simulink model "test_SYSTEME_ZIGBEE_2017"  (R2014b)
settings: Solver=ode45  SolverMode=SingleTasking  StartTime=0.0  StopTime=1E-3  RelTol=1e-3
libraries: dspsrcs4 x8, dsparch4 x7, simulink x3, dspstat3 x2, commsink2 x1, commrandsrc2 x1, commdigbbndcpm2 x1, simulink_extras x1, dspsigops x1
settings Model: DisableUpgradeWarningsForVersion=R2015a  CovSFcnEnable=on  Creator=Yannis  LastModifiedBy=xph2app003
settings OptimizationCC: BlockReduction=off  BooleanDataType=off
settings DebuggingCC: SaveWithParameterizedLinksMsg=none  UnderspecifiedInitializationDetection=Classic  MergeDetectMultiDrivingBlocksExec=none  SignalResolutionControl=TryResolveAllWithWarning  SolverPrmCheckMsg=none
settings HardwareCC: TargetBitPerLong=64  TargetBitPerPointer=64  TargetLongLongMode=on  TargetIntDivRoundTo=Zero  TargetEndianess=LittleEndian  TargetWordSize=64  TargetHWDeviceType=MATLAB Host  ProdEqTarget=off

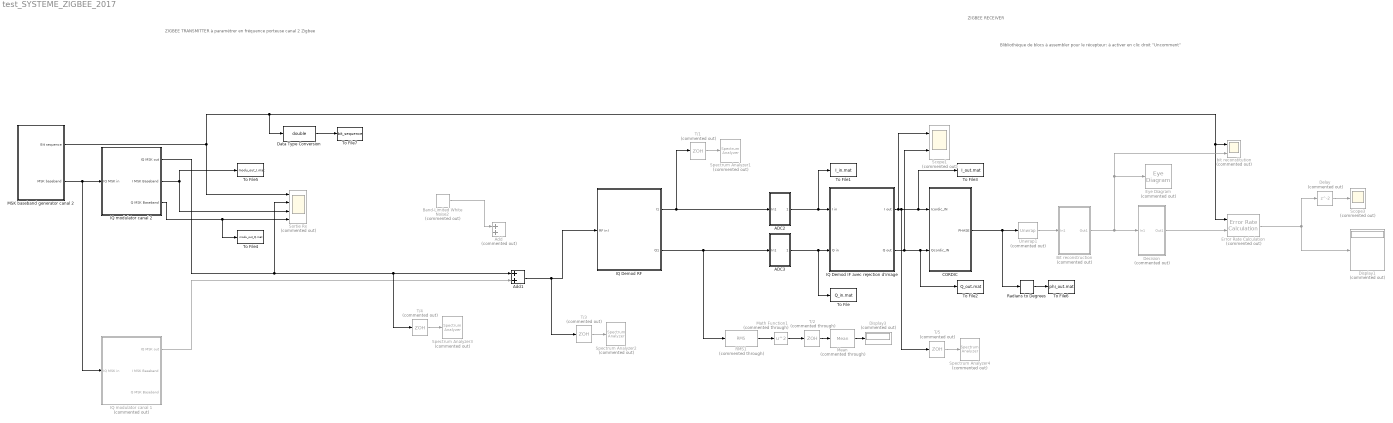
== system test_SYSTEME_ZIGBEE_2017 ==
  note: ZIGBEE RECEIVER
  note: ZIGBEE TRANSMITTER
      | à paramétrer en fréquence porteuse
      | canal 2  Zigbee
  note: Blibliothèque de blocs à assembler pour le récepteur: à activer en clic droit "Uncomment"
  ADC2 : Subsystem
  ADC3 : Subsystem
  Add : Sum  Commented=on
  Add1 : Sum
  Band-Limited White Noise2 : simulink/Sources/Band-Limited White Noise  Commented=on  Cov=[1e-9]  Ts=5e-10  seed=[23341]
  Bit reconstruction : Subsystem  Commented=on
  CORDIC : Subsystem
  Data Type Conversion : DataTypeConversion  OutDataTypeStr=double
  Decision : Subsystem  Commented=on
  Delay : Delay  Commented=on  InitialCondition=0
  Display1 : Display  Commented=on
  Display3 : Display  Commented=on
  Error Rate Calculation : commsink2/Error Rate Calculation  Commented=on  N=1  st_delay=1  cp_mode=Entire frame  subframe=[]  PMode=Port  WsName=ErrorVec  RsMode2=off  stop=off  numErr=100  maxBits=1e6
  Eye Diagram : EyeDiagram  Commented=on
  IQ Demod IF avec rejection d'image : Subsystem  TreatAsAtomicUnit=on
  IQ Demod RF : Subsystem  TreatAsAtomicUnit=on
  IQ modulator canal 1 : Subsystem  Commented=on
  IQ modulator canal 2 : Subsystem
  MSK baseband generator canal 2 : Subsystem
  Math Function1 : Math  Commented=through  Operator=square  SaturateOnIntegerOverflow=on
  Mean : dspstat3/Mean  Commented=through  run=on  reset_popup=None  InputProcessing=Columns as channels (frame based)  directionMode=Each column  dimension=1  treatSBRowAsCol=on  roiEnable=off  roiType=Rectangles  roiPortion=Entire ROI  roiOutput=Individual statistics for each ROI  roiFlag=off  outputDataTypeStr=Inherit: Same as accumulator  outputLastDataTypeStr=Inherit: Same as accumulator  outputMin=[]  outputMax=[]  roundingMode=Floor  overflowMode=off
  RMS1 : dspstat3/RMS  Commented=through  run=off  reset_popup=None  InputProcessing=Columns as channels (frame based)  directionMode=Entire input  dimension=1  treatSBRowAsCol=on
  Radians to Degrees : simulink_extras/Transformations/Radians to Degrees
  Scope1 : Scope  Commented=on  NumInputPorts=2
      settings: YMin=-1.5~-1.5  YMax=1.5~1.5  MaxDataPoints=20000
  Scope3 : Scope  Commented=on
      settings: TimeRange=9.999999999999999e-05  YMin=-1  YMax=1  SaveName=ScopeData2
  Sortie Rx : Scope  Commented=on  NumInputPorts=4
      settings: TimeRange=1e-05  YMin=-1~-1.5~-1~-1  YMax=2~1.5~1~1
  Spectrum Analyzer{1..4} (4 alike) : SpectrumAnalyzer  Commented=on
  T/{1,3..5} (4 alike) : ZeroOrderHold  Commented=on  SampleTime=1/(10e6)
  T/2 : ZeroOrderHold  Commented=through  SampleTime=1/(10e6)
  To File : ToFile  Filename=Q_in.mat
  To File1 : ToFile  Filename=I_in.mat
  To File2 : ToFile  Filename=Q_out.mat
  To File3 : ToFile  Filename=I_out.mat
  To File4 : ToFile  Filename=modu_out_Q.mat
  To File5 : ToFile  Filename=modu_out_I.mat
  To File6 : ToFile  Filename=phi_out.mat
  To File7 : ToFile  Filename=bit_sequence  MatrixName=bit
  Unwrap1 : dspsigops/Unwrap  Commented=on  tol=pi  InputProcessing=Columns as channels (frame based)  running=off
  bit reconstitution : Scope  Commented=on  NumInputPorts=2
      settings: TimeRange=1.049040685224839e-05  YMin=-0.2~-2  YMax=3~0.6  SaveName=ScopeData4
  wires:
  Delay/1 -> Scope3/1
  MSK baseband generator canal 2/1(Bit sequence) -> Data Type Conversion/1, Error Rate Calculation/1, bit reconstitution/1, Sortie Rx/1
  IQ modulator canal 2/3(Q MSK Baseband) -> To File4/1, Sortie Rx/4
  Error Rate Calculation/1 -> Display1/1, Delay/1
  ADC2/1(Out1) -> To File1/1, IQ Demod IF avec rejection d'image/1("I in ")
  ADC3/1(Out1) -> To File/1, IQ Demod IF avec rejection d'image/2("Q in ")
  IQ modulator canal 2/2(I MSK Baseband) -> Sortie Rx/3, To File5/1
  IQ Demod RF/1(I1) -> ADC2/1(In1), T/1/1
  IQ Demod RF/2("Q1 ") -> RMS1/1, ADC3/1(In1)
  IQ Demod IF avec rejection d'image/2(Q out) -> To File2/1, CORDIC/2(Qcordic_IN), Scope1/2
  CORDIC/1(PHASE) -> Radians to Degrees/1, Unwrap1/1
  Unwrap1/1 -> Bit reconstruction/1(In1)
  Bit reconstruction/1(Out1) -> Eye Diagram/1, bit reconstitution/2, Decision/1(In1)
  T/1/1 -> Spectrum Analyzer1/1
  Decision/1(Out1) -> Error Rate Calculation/2
  Band-Limited White Noise2/1 -> Add/1
  RMS1/1 -> Math Function1/1
  T/2/1 -> Mean/1
  Mean/1 -> Display3/1
  Math Function1/1 -> T/2/1
  MSK baseband generator canal 2/2(MSK baseband) -> IQ modulator canal 1/1(IQ MSK in), IQ modulator canal 2/1(IQ MSK in)
  IQ modulator canal 1/1("IQ MSK out ") -> Add1/2
  Add1/1 -> T/3/1, IQ Demod RF/1(RF in I)
  T/3/1 -> Spectrum Analyzer2/1
  IQ modulator canal 2/1("IQ MSK out ") -> Sortie Rx/2, T/4/1, Add1/1
  T/4/1 -> Spectrum Analyzer3/1
  IQ Demod IF avec rejection d'image/1(I out) -> To File3/1, CORDIC/1(Icordic_IN), T/5/1, Scope1/1
  T/5/1 -> Spectrum Analyzer4/1
  Data Type Conversion/1 -> To File7/1
  Radians to Degrees/1 -> To File6/1

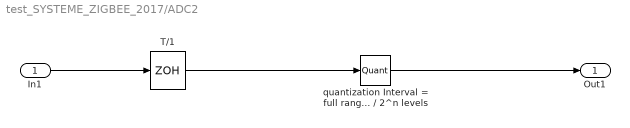
== system test_SYSTEME_ZIGBEE_2017/ADC2 ==
  In1 : Inport
  T/1 : ZeroOrderHold  SampleTime=1/(50e6)
  quantization Interval = full range (2Volts) / 2^n levels : Quantizer  QuantizationInterval=2/32  LinearizeAsGain=off  SampleTime=1/(50e6)
  Out1 : Outport
  wires:
  In1/1 -> T/1/1
  T/1/1 -> quantization Interval = full range (2Volts) / 2^n levels/1
  quantization Interval = full range (2Volts) / 2^n levels/1 -> Out1/1

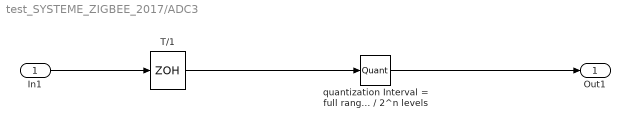
== system test_SYSTEME_ZIGBEE_2017/ADC3 ==
  In1 : Inport
  T/1 : ZeroOrderHold  SampleTime=1/(50e6)
  quantization Interval = full range (2Volts) / 2^n levels : Quantizer  QuantizationInterval=2/32  LinearizeAsGain=off  SampleTime=1/(50e6)
  Out1 : Outport
  wires:
  In1/1 -> T/1/1
  T/1/1 -> quantization Interval = full range (2Volts) / 2^n levels/1
  quantization Interval = full range (2Volts) / 2^n levels/1 -> Out1/1

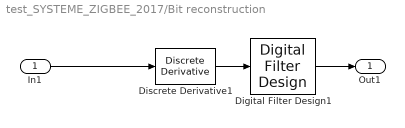
== system test_SYSTEME_ZIGBEE_2017/Bit reconstruction ==
  In1 : Inport
  Digital Filter Design1 : dsparch4/Digital Filter Design  mwdsp_browser_bugfix_var=off
  Discrete Derivative1 : simulink/Discrete/Discrete Derivative  gainval=1/(10e6)  ICPrevScaledInput=0.0  InputProcessing=Inherited  OutMin=[]  OutMax=[]  OutDataTypeStr=double  OutputDataTypeScalingMode=double  OutDataType=fixdt(1, 16)  OutScaling=2^-10  DoSatur=off
  Out1 : Outport
  wires:
  Discrete Derivative1/1 -> Digital Filter Design1/1
  Digital Filter Design1/1 -> Out1/1
  In1/1 -> Discrete Derivative1/1

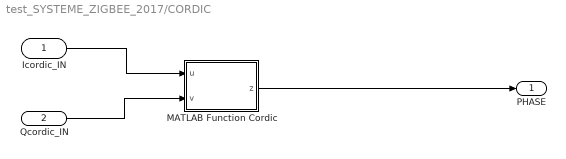
== system test_SYSTEME_ZIGBEE_2017/CORDIC ==
  Icordic_IN : Inport
  Qcordic_IN : Inport  Port=2
  MATLAB Function Cordic : MATLAB Function  TreatAsAtomicUnit=on
  PHASE : Outport
  wires:
  MATLAB Function Cordic/1(z) -> PHASE/1
  Icordic_IN/1 -> MATLAB Function Cordic/1(u)
  Qcordic_IN/1 -> MATLAB Function Cordic/2(v)

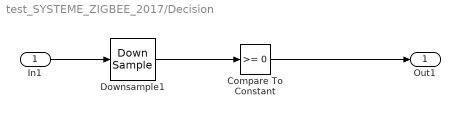
== system test_SYSTEME_ZIGBEE_2017/Decision ==
  In1 : Inport
  Compare To Constant : simulink/Logic and Bit Operations/Compare To Constant  relop=>=  const=0  OutDataTypeStr=boolean
  Downsample1 : DownSample  N=5  phase=2
  Out1 : Outport
  wires:
  Compare To Constant/1 -> Out1/1
  In1/1 -> Downsample1/1
  Downsample1/1 -> Compare To Constant/1

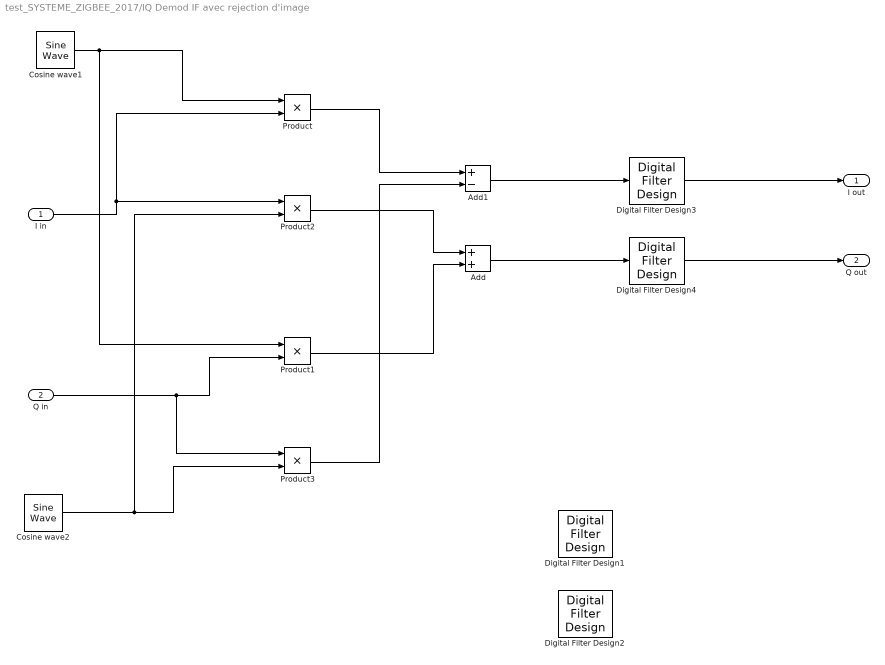
== system test_SYSTEME_ZIGBEE_2017/IQ Demod IF avec rejection d'image ==
  "I in " : Inport
  "Q in " : Inport  Port=2
  Add : Sum
  Add1 : Sum  Inputs=+-
  Cosine wave1 : dspsrcs4/Sine Wave  Amplitude=1  Frequency=2.5e6  Phase=pi/2  SampleMode=Discrete  OutComplex=Real  CompMethod=Trigonometric fcn  TableSize=Speed  SampleTime=1/(50e6)  SamplesPerFrame=1  ResetState=Restart at time zero  dataType=double  wordLen=16  udDataType=sfix(16)  fracBitsMode=Best precision  numFracBits=15  OutDataTypeStr=double  LastOutDataTypeStr=double
  Cosine wave2 : dspsrcs4/Sine Wave  Amplitude=1  Frequency=2.5e6  Phase=pi  SampleMode=Discrete  OutComplex=Real  CompMethod=Trigonometric fcn  TableSize=Speed  SampleTime=1/(50e6)  SamplesPerFrame=1  ResetState=Restart at time zero  dataType=double  wordLen=16  udDataType=sfix(16)  fracBitsMode=Best precision  numFracBits=15  OutDataTypeStr=double  LastOutDataTypeStr=double
  Digital Filter Design{1..4} (4 alike) : dsparch4/Digital Filter Design  mwdsp_browser_bugfix_var=off
  Product{,1..3} (4 alike) : Product
  I out : Outport
  Q out : Outport  Port=2
  wires:
  Cosine wave1/1 -> Product1/1, Product/1
  Cosine wave2/1 -> Product2/2, Product3/2
  "I in "/1 -> Product2/1, Product/2
  "Q in "/1 -> Product3/1, Product1/2
  Product/1 -> Add1/1
  Product3/1 -> Add1/2
  Product2/1 -> Add/1
  Product1/1 -> Add/2
  Add/1 -> Digital Filter Design4/1
  Digital Filter Design4/1 -> Q out/1
  Digital Filter Design3/1 -> I out/1
  Add1/1 -> Digital Filter Design3/1

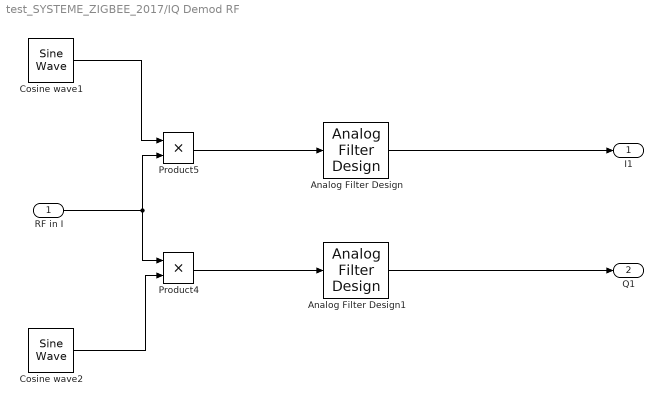
== system test_SYSTEME_ZIGBEE_2017/IQ Demod RF ==
  RF in I : Inport
  Analog Filter Design : dsparch4/Analog Filter Design  method=Butterworth  filttype=Lowpass  N=8  Wlo=31.4e6  Whi=80  Rp=2  Rs=40
  Analog Filter Design1 : dsparch4/Analog Filter Design  method=Butterworth  filttype=Lowpass  N=8  Wlo=31.4e6  Whi=80  Rp=2  Rs=40
  Cosine wave1 : dspsrcs4/Sine Wave  Amplitude=1  Frequency=2.4075e9  Phase=pi/2  SampleMode=Continuous  OutComplex=Real  CompMethod=Trigonometric fcn  TableSize=Speed  SampleTime=1/(10e6)  SamplesPerFrame=1  ResetState=Restart at time zero  dataType=double  wordLen=16  udDataType=sfix(16)  fracBitsMode=Best precision  numFracBits=15  OutDataTypeStr=double  LastOutDataTypeStr=double
  Cosine wave2 : dspsrcs4/Sine Wave  Amplitude=1  Frequency=2.4075e9  Phase=pi  SampleMode=Continuous  OutComplex=Real  CompMethod=Trigonometric fcn  TableSize=Speed  SampleTime=1/(10e6)  SamplesPerFrame=1  ResetState=Restart at time zero  dataType=double  wordLen=16  udDataType=sfix(16)  fracBitsMode=Best precision  numFracBits=15  OutDataTypeStr=double  LastOutDataTypeStr=double
  Product4 : Product  RndMeth=Zero
  Product5 : Product  RndMeth=Zero
  I1 : Outport
  "Q1 " : Outport  Port=2
  wires:
  RF in I/1 -> Product5/2, Product4/1
  Cosine wave2/1 -> Product4/2
  Cosine wave1/1 -> Product5/1
  Product5/1 -> Analog Filter Design/1
  Product4/1 -> Analog Filter Design1/1
  Analog Filter Design/1 -> I1/1
  Analog Filter Design1/1 -> "Q1 "/1

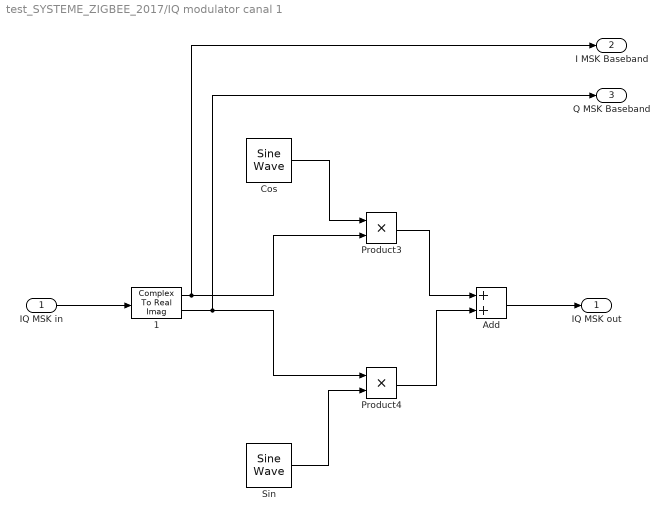
== system test_SYSTEME_ZIGBEE_2017/IQ modulator canal 1 ==
  IQ MSK in : Inport
  " 1" : ComplexToRealImag
  Add : Sum
  Cos : dspsrcs4/Sine Wave  Amplitude=1  Frequency=2.405e9  Phase=pi/2  SampleMode=Continuous  OutComplex=Real  CompMethod=Trigonometric fcn  TableSize=Speed  SampleTime=1/(8*2.4e9)  SamplesPerFrame=1  ResetState=Restart at time zero  dataType=double  wordLen=16  udDataType=sfix(16)  fracBitsMode=Best precision  numFracBits=15  OutDataTypeStr=double  LastOutDataTypeStr=double
  Product3 : Product  RndMeth=Zero
  Product4 : Product  RndMeth=Zero
  Sin : dspsrcs4/Sine Wave  Amplitude=1  Frequency=2.405E9  Phase=pi  SampleMode=Continuous  OutComplex=Real  CompMethod=Trigonometric fcn  TableSize=Speed  SampleTime=1/(4*2.4e9)  SamplesPerFrame=1  ResetState=Restart at time zero  dataType=double  wordLen=16  udDataType=sfix(16)  fracBitsMode=Best precision  numFracBits=15  OutDataTypeStr=double  LastOutDataTypeStr=double
  "IQ MSK out " : Outport
  I MSK Baseband : Outport  Port=2
  Q MSK Baseband : Outport  Port=3
  wires:
  Add/1 -> "IQ MSK out "/1
  Product4/1 -> Add/2
  " 1"/2 -> Product4/1, Q MSK Baseband/1
  " 1"/1 -> I MSK Baseband/1, Product3/2
  Sin/1 -> Product4/2
  Product3/1 -> Add/1
  Cos/1 -> Product3/1
  IQ MSK in/1 -> " 1"/1

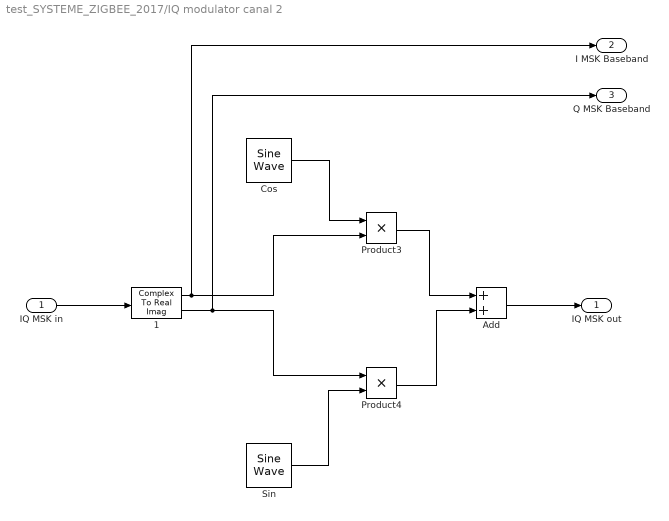
== system test_SYSTEME_ZIGBEE_2017/IQ modulator canal 2 ==
  IQ MSK in : Inport
  " 1" : ComplexToRealImag
  Add : Sum
  Cos : dspsrcs4/Sine Wave  Amplitude=1  Frequency=2.410e9  Phase=pi/2  SampleMode=Continuous  OutComplex=Real  CompMethod=Trigonometric fcn  TableSize=Speed  SampleTime=1/(8*2.4e9)  SamplesPerFrame=1  ResetState=Restart at time zero  dataType=double  wordLen=16  udDataType=sfix(16)  fracBitsMode=Best precision  numFracBits=15  OutDataTypeStr=double  LastOutDataTypeStr=double
  Product3 : Product  RndMeth=Zero
  Product4 : Product  RndMeth=Zero
  Sin : dspsrcs4/Sine Wave  Amplitude=1  Frequency=2.410E9  Phase=pi  SampleMode=Continuous  OutComplex=Real  CompMethod=Trigonometric fcn  TableSize=Speed  SampleTime=1/(4*2.4e9)  SamplesPerFrame=1  ResetState=Restart at time zero  dataType=double  wordLen=16  udDataType=sfix(16)  fracBitsMode=Best precision  numFracBits=15  OutDataTypeStr=double  LastOutDataTypeStr=double
  "IQ MSK out " : Outport
  I MSK Baseband : Outport  Port=2
  Q MSK Baseband : Outport  Port=3
  wires:
  Add/1 -> "IQ MSK out "/1
  Product4/1 -> Add/2
  " 1"/2 -> Product4/1, Q MSK Baseband/1
  " 1"/1 -> I MSK Baseband/1, Product3/2
  Sin/1 -> Product4/2
  Product3/1 -> Add/1
  Cos/1 -> Product3/1
  IQ MSK in/1 -> " 1"/1

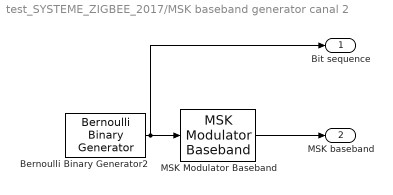
== system test_SYSTEME_ZIGBEE_2017/MSK baseband generator canal 2 ==
  Bernoulli Binary Generator2 : commrandsrc2/Bernoulli Binary Generator  P=0.5  seed=0  Ts=0.5e-6  frameBased=off  sampPerFrame=1  orient=off  outDataType=boolean
  MSK Modulator Baseband : commdigbbndcpm2/MSK Modulator Baseband  inputType=Bit  phaseOffset=0  samplesPerSymbol=20  RateOptions=Inherit from input (this choice will be removed - see release notes)  outDataType=double
  Bit sequence : Outport
  MSK baseband : Outport  Port=2
  wires:
  Bernoulli Binary Generator2/1 -> Bit sequence/1, MSK Modulator Baseband/1
  MSK Modulator Baseband/1 -> MSK baseband/1

== matlab function test_SYSTEME_ZIGBEE_2017/CORDIC/MATLAB Function Cordic ==
  data: u input; z output; v input
function z = fcn(u,v)
%#codegen

I0=u;
Q0=v;
I=zeros(1,9);
Q=zeros(1,9);
I(1)=u;
Q(1)=v;
k=0;
z=0;
c1=0;
c2=0;


if I0<0
    if Q0>0
    I(1)=-I0;
    Q(1)=-Q0;
    c1=1;
    end
    if Q0<0
    I(1)=-I0;
    Q(1)=-Q0;
    c2=1;
    end
end

if  I0==0
    if Q0<0;
        z=-pi/2;
    end
    if Q0>0
        z=+pi/2;
    end
end


    
if I(1)>0
    while (k<8)
        if Q(k+1)<0
        Q(k+2)=Q(k+1)+I(k+1)*2^(-k);
        I(k+2)=I(k+1)-Q(k+1)*2^(-k);
        z=z-atan(2^(-(k)));
        end
        if Q(k+1)>0
        Q(k+2)=Q(k+1)-I(k+1)*2^(-k);
        I(k+2)=I(k+1)+Q(k+1)*2^(-k);
        z=z+atan(2^(-k));
        end
        if Q(k+1)==0
        break;
        end
        k=k+1;
    end

end

if c1==1
    z=pi+z;
end

if c2==1
    z=-pi+z;
end

 
end
